simulink model "battery"  (R2023b)
settings: Solver=VariableStepAuto  StartTime=0.0  StopTime=inf  FixedStep=0.01  RelTol=1e-3
model workspace (MAT data in the model file):
  AH = Simulink.Parameter
  AH.Value = 3
  AH.DataType = 'auto'
  AH.Complexity = 'real'
  AH.Dimensions = [1 1]
  R0 = Simulink.Parameter
  R0.Value = 0.003
  R0.DataType = 'auto'
  R0.Complexity = 'real'
  R0.Dimensions = [1 1]
libraries: BatteryEstimators x1
settings Model: PacingRate=100  Creator=chris  LastModifiedBy=chris

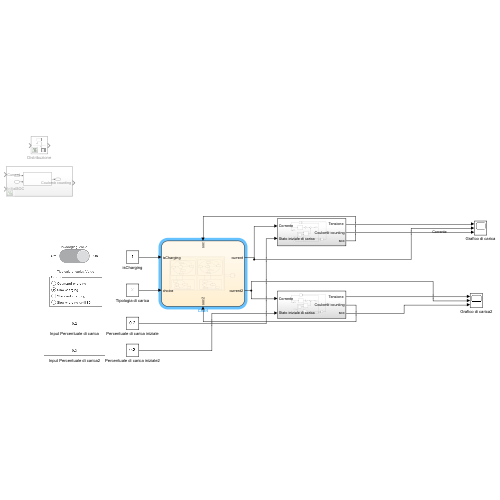
[thumbnail: Simulink's stored preview of the top-level diagram]
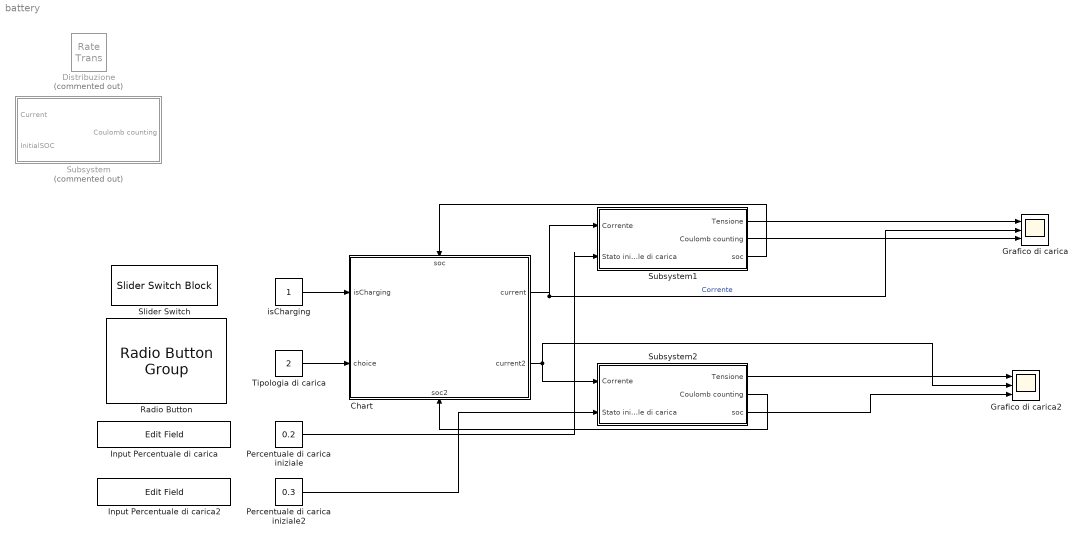
== system battery ==
  Chart : Stateflow chart  TreatAsAtomicUnit=on
      settings: PortSchema="{\"entries\":[{\"content\":{\"sides\":[{\"content\":{\"connectorIds\":[\"In1\",\"In3\"]},\"type\":\"ConnectorPlacement.EquallySpacedRectSide\",\"uuid\":\"a6672bef-1ba0-496b-9c5e-64820f88021e\"},{\"content\":{\"connectorIds\":[\"Out1\",\"Out2\"],\"side\":\"RIGHT\"},\"type\":\"ConnectorPlacement.EquallySpacedRectSide\",\"uuid\":\"9e4eb33c-d745-4260-a0dc-36479670b9dc\"},{\"content\":{\"connectorIds\":[\"In2\"],\"side\":\"TOP\"},\"type\":\"ConnectorPlacement.EquallySpacedRectSide\",\"uuid\":\"ece41cf9-1d3b-45f4-8ae6-354b3a498270\"},{\"content\":{\"connectorIds\":[\"In4\"],\"side\":\"BOTTOM\"},\"type\":\"ConnectorPlacement.EquallySpacedRectSide\",\"uuid\":\"edd66967-5ff2-47ba-bdfe-f7b79a318669\"}]},\"type\":\"ConnectorPlacement.EquallySpacedConnector\",\"uuid\":\"4cccf6ba-1acf-421a-acb7-d2646cbad516\"}],\"packageUris\":[\"http://schema.mathworks.com/mf0/Connector/R2020b\"],\"version\":\"1.0\"}"
  Distribuzione : RateTransition  Commented=on  InitialCondition=0.1
  Grafico di carica : Scope  NumInputPorts=3
  Grafico di carica2 : Scope  NumInputPorts=3
  Input Percentuale di carica : EditField  LabelPosition=Hide  ShowInitialText=on  Alignment=Center
  Input Percentuale di carica2 : EditField  LabelPosition=Hide  ShowInitialText=on  Alignment=Center
  Percentuale di carica iniziale : Constant  Value=0.2
  Percentuale di carica iniziale2 : Constant  Value=0.3
  Radio Button : RadioButtonGroup  SelectedLabel=Slow charging  ButtonGroupName=Group
      settings: Values={{'Optimized charging', 'Slow charging', 'Standard charging', 'Slow charging until 80'}, [1 2 3 4]}
  Slider Switch : SliderSwitchBlock
      settings: Values={{'Off', 'On'}, [0 1]}
  Subsystem : Subsystem  Commented=on
  Subsystem1 : Subsystem
  Subsystem2 : Subsystem
  Tipologia di carica : Constant  Value=2
  isCharging : Constant
  wires:
  Tipologia di carica/1 -> Chart/3(choice)
  isCharging/1 -> Chart/1(isCharging)
  Chart/1(current) -> Subsystem1/1(Corrente), Grafico di carica/2  "Corrente"
  Percentuale di carica iniziale/1 -> Subsystem1/2(Stato iniziale di carica)
  Subsystem1/1("Tensione ") -> Grafico di carica/1
  Subsystem1/2(Coulomb counting) -> Grafico di carica/3
  Subsystem1/3(soc) -> Chart/2(soc)
  Percentuale di carica iniziale2/1 -> Subsystem2/2(Stato iniziale di carica)
  Chart/2(current2) -> Subsystem2/1(Corrente), Grafico di carica2/2
  Subsystem2/3(soc) -> Grafico di carica2/3
  Subsystem2/1("Tensione ") -> Grafico di carica2/1
  Subsystem2/2(Coulomb counting) -> Chart/4(soc2)

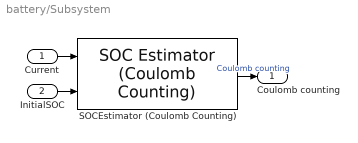
== system battery/Subsystem ==
  Current : Inport
  InitialSOC : Inport  Port=2
  SOCEstimator (Coulomb Counting) : BatteryEstimators/SOC Estimator (Coulomb Counting)  CurrentInputPartition=off  AH=3  Ts=2
      settings: LibrarySourceBlock=|
      | batt_sl_lib/Estimators/SOC Estimator
      | (Coulomb Counting)
  Coulomb counting : Outport
  wires:
  SOCEstimator (Coulomb Counting)/1 -> Coulomb counting/1  "Coulomb counting"
  InitialSOC/1 -> SOCEstimator (Coulomb Counting)/2
  Current/1 -> SOCEstimator (Coulomb Counting)/1

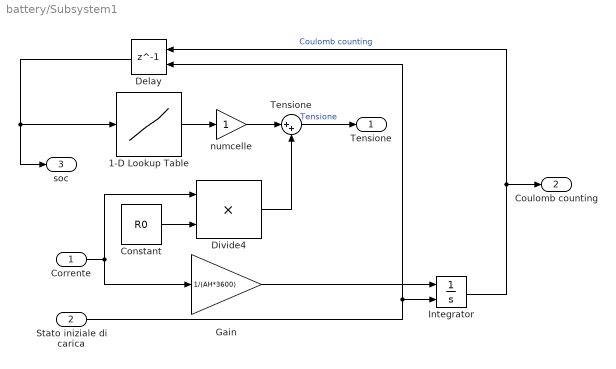
== system battery/Subsystem1 ==
  Corrente : Inport
  Stato iniziale di carica : Inport  Port=2
  1-D Lookup Table : Lookup_n-D  NumberOfTableDimensions=1  BreakpointsForDimension1=[0, .1, .38,.511,.8,.92, 1]  Table=[3.28, 3.45, 3.63, 3.69,3.95,4.01,4.2]  InternalRulePriority=Speed  RndMeth=Simplest
  Constant : Constant  Value=R0
  Delay : Delay  DelayLength=1  InitialConditionSource=Input port
      settings: InputPortMap=u0,p4
  Divide4 : Product  Inputs=**
  Gain : Gain  Gain=1/(AH*3600)
  Integrator : Integrator  InitialConditionSource=external
  Tensione : Sum  Inputs=|++
  numcelle : Gain
  "Tensione " : Outport
  Coulomb counting : Outport  Port=2
  soc : Outport  Port=3
  wires:
  Divide4/1 -> Tensione/2
  Corrente/1 -> Divide4/1, Gain/1
  Delay/1 -> soc/1, 1-D Lookup Table/1
  Stato iniziale di carica/1 -> Delay/2, Integrator/2
  numcelle/1 -> Tensione/1
  Gain/1 -> Integrator/1
  Constant/1 -> Divide4/2
  1-D Lookup Table/1 -> numcelle/1
  Integrator/1 -> Delay/1, Coulomb counting/1  "Coulomb counting"
  Tensione/1 -> "Tensione "/1  "Tensione"

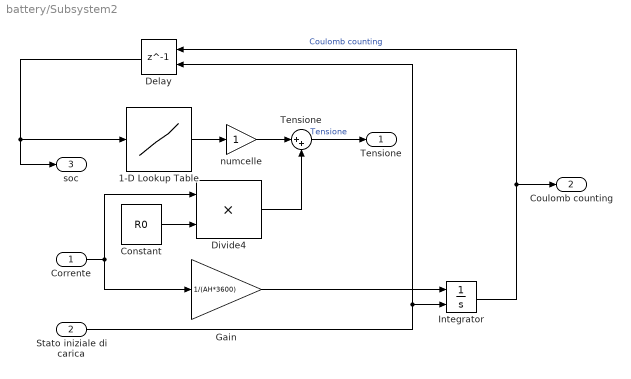
== system battery/Subsystem2 ==
  Corrente : Inport
  Stato iniziale di carica : Inport  Port=2
  1-D Lookup Table : Lookup_n-D  NumberOfTableDimensions=1  BreakpointsForDimension1=[0, .1, .38,.511,.8,.92, 1]  Table=[3.28, 3.45, 3.63, 3.69,3.95,4.01,4.2]  InternalRulePriority=Speed  RndMeth=Simplest
  Constant : Constant  Value=R0
  Delay : Delay  DelayLength=1  InitialConditionSource=Input port
      settings: InputPortMap=u0,p4
  Divide4 : Product  Inputs=**
  Gain : Gain  Gain=1/(AH*3600)
  Integrator : Integrator  InitialConditionSource=external
  Tensione : Sum  Inputs=|++
  numcelle : Gain
  "Tensione " : Outport
  Coulomb counting : Outport  Port=2
  soc : Outport  Port=3
  wires:
  Divide4/1 -> Tensione/2
  Corrente/1 -> Divide4/1, Gain/1
  Delay/1 -> soc/1, 1-D Lookup Table/1
  Stato iniziale di carica/1 -> Delay/2, Integrator/2
  numcelle/1 -> Tensione/1
  Gain/1 -> Integrator/1
  Constant/1 -> Divide4/2
  1-D Lookup Table/1 -> numcelle/1
  Integrator/1 -> Delay/1, Coulomb counting/1  "Coulomb counting"
  Tensione/1 -> "Tensione "/1  "Tensione"

== stateflow chart battery/Chart ==
  settings: updateMethod=CONTINUOUS  sampleTime=1
  state BatteryOn
    state BatteryOn2 [parallel]
      settings: executionOrder=2
      state Charging
        state FastCharge
          en: current2 = 3
        state SlowCharge
          en: current2 = 1
        state gest1
        state regular
          en: current2 = 1.5
        state slowChargeuntil80
          en: current2 = 1
        state idle
          en: current2 = 0
        BatteryOn.BatteryOn2.Charging.regular -> BatteryOn.BatteryOn2.Charging.SlowCharge [order 2] : [soc2 >= 0.5]
        BatteryOn.BatteryOn2.Charging.FastCharge -> BatteryOn.BatteryOn2.Charging.SlowCharge : [soc2 >= 0.7]
        BatteryOn.BatteryOn2.Charging.gest1 -> BatteryOn.BatteryOn2.Charging.FastCharge [order 1] : [choice == 1]
        (default) -> BatteryOn.BatteryOn2.Charging.gest1
        BatteryOn.BatteryOn2.Charging.gest1 -> BatteryOn.BatteryOn2.Charging.SlowCharge [order 2] : [choice ==2]
        BatteryOn.BatteryOn2.Charging.gest1 -> BatteryOn.BatteryOn2.Charging.regular [order 3] : [choice == 3]
        BatteryOn.BatteryOn2.Charging.SlowCharge -> BatteryOn.BatteryOn2.Charging.idle : [soc2>=0.98]
        BatteryOn.BatteryOn2.Charging.regular -> BatteryOn.BatteryOn2.Charging.idle [order 1] : [soc2 >=0.98]
        BatteryOn.BatteryOn2.Charging.gest1 -> BatteryOn.BatteryOn2.Charging.idle [order 5] : [soc2>=0.98]
        BatteryOn.BatteryOn2.Charging.gest1 -> BatteryOn.BatteryOn2.Charging.slowChargeuntil80 [order 4] : [choice == 4]
        BatteryOn.BatteryOn2.Charging.slowChargeuntil80 -> BatteryOn.BatteryOn2.Charging.idle : [soc2 >= 0.78]
      note: corrente negativa sarebbe consumo di corrente
      state Discharging
        state PerformanceMode
          en: current2 = - 3
        state normalmode
          en: current2 = - 1.5
        state Manager
        state idle
          en: current2 = 0
        state BatterySaverMode
          en: current2 = - 1
        BatteryOn.BatteryOn2.Discharging.PerformanceMode -> BatteryOn.BatteryOn2.Discharging.normalmode : [soc2 < 0.5]
        BatteryOn.BatteryOn2.Discharging.Manager -> BatteryOn.BatteryOn2.Discharging.PerformanceMode [order 2] : [soc2 >= 0.8]
        BatteryOn.BatteryOn2.Discharging.Manager -> BatteryOn.BatteryOn2.Discharging.normalmode [order 1] : [soc2 > 0.2 & soc2 < 0.8]
        (default) -> BatteryOn.BatteryOn2.Discharging.Manager
        BatteryOn.BatteryOn2.Discharging.normalmode -> BatteryOn.BatteryOn2.Discharging.BatterySaverMode : [soc2 < 0.2]
        BatteryOn.BatteryOn2.Discharging.Manager -> BatteryOn.BatteryOn2.Discharging.BatterySaverMode [order 3] : [soc2 <= 0.2 ]
        BatteryOn.BatteryOn2.Discharging.BatterySaverMode -> BatteryOn.BatteryOn2.Discharging.idle : [soc2<=0.01]
      (default) -> BatteryOn.BatteryOn2.Charging
      BatteryOn.BatteryOn2.Charging -> BatteryOn.BatteryOn2.Discharging : [isCharging == 0]
      BatteryOn.BatteryOn2.Discharging -> BatteryOn.BatteryOn2.Charging : [isCharging == 1 ]
    state BatteryOn1 [parallel]
      settings: executionOrder=1
      state Charging
        state FastCharge
          en: current = 3
        state SlowCharge
          en: current = 1
        state gest1
        state regular
          en: current = 1.5
        state slowChargeuntil80
          en: current = 1
        state idle
          en: current = 0
        BatteryOn.BatteryOn1.Charging.regular -> BatteryOn.BatteryOn1.Charging.SlowCharge [order 2] : [soc >= 0.5]
        BatteryOn.BatteryOn1.Charging.FastCharge -> BatteryOn.BatteryOn1.Charging.SlowCharge : [soc >= 0.7]
        BatteryOn.BatteryOn1.Charging.gest1 -> BatteryOn.BatteryOn1.Charging.FastCharge [order 1] : [choice == 1]
        (default) -> BatteryOn.BatteryOn1.Charging.gest1
        BatteryOn.BatteryOn1.Charging.gest1 -> BatteryOn.BatteryOn1.Charging.SlowCharge [order 2] : [choice ==2]
        BatteryOn.BatteryOn1.Charging.gest1 -> BatteryOn.BatteryOn1.Charging.regular [order 3] : [choice == 3]
        BatteryOn.BatteryOn1.Charging.SlowCharge -> BatteryOn.BatteryOn1.Charging.idle : [soc>=0.98]
        BatteryOn.BatteryOn1.Charging.regular -> BatteryOn.BatteryOn1.Charging.idle [order 1] : [soc>=0.98]
        BatteryOn.BatteryOn1.Charging.gest1 -> BatteryOn.BatteryOn1.Charging.idle [order 5] : [soc>=0.98]
        BatteryOn.BatteryOn1.Charging.gest1 -> BatteryOn.BatteryOn1.Charging.slowChargeuntil80 [order 4] : [choice == 4]
        BatteryOn.BatteryOn1.Charging.slowChargeuntil80 -> BatteryOn.BatteryOn1.Charging.idle : [soc >= 0.78]
      note: corrente negativa sarebbe consumo di corrente
      state Discharging
        state PerformanceMode
          en: current = - 3
        state Manager
        state normalmode
          en: current = - 1.5
        state idle
          en: current = 0
        state BatterySaverMode
          en: current = - 1
        BatteryOn.BatteryOn1.Discharging.PerformanceMode -> BatteryOn.BatteryOn1.Discharging.normalmode : [soc < 0.5]
        BatteryOn.BatteryOn1.Discharging.Manager -> BatteryOn.BatteryOn1.Discharging.PerformanceMode [order 2] : [soc >= 0.8]
        BatteryOn.BatteryOn1.Discharging.Manager -> BatteryOn.BatteryOn1.Discharging.normalmode [order 1] : [soc > 0.2 & soc < 0.8]
        (default) -> BatteryOn.BatteryOn1.Discharging.Manager
        BatteryOn.BatteryOn1.Discharging.normalmode -> BatteryOn.BatteryOn1.Discharging.BatterySaverMode : [soc < 0.2]
        BatteryOn.BatteryOn1.Discharging.Manager -> BatteryOn.BatteryOn1.Discharging.BatterySaverMode [order 3] : [soc <= 0.2 ]
        BatteryOn.BatteryOn1.Discharging.BatterySaverMode -> BatteryOn.BatteryOn1.Discharging.idle : [soc<=0.01]
      (default) -> BatteryOn.BatteryOn1.Charging
      BatteryOn.BatteryOn1.Charging -> BatteryOn.BatteryOn1.Discharging : [isCharging == 0]
      BatteryOn.BatteryOn1.Discharging -> BatteryOn.BatteryOn1.Charging : [isCharging == 1 ]
  state Batteryoff
    en: current = 0
    current2 = 0
  Batteryoff -> BatteryOn : [isCharging == 1|| soc>0.01 || soc2 > 0.01]
  (default) -> Batteryoff
  BatteryOn -> Batteryoff : [soc2<=0.01 && soc<=0.01 && isCharging == 0]
  data: isCharging input; current output =0; soc input; choice input; soc2 input; current2 output
  data current settings: updateMethod=SF_CONTINUOUS_TIME_DATA
